simulink model "arch_logical"  (R2026a)
settings: Solver=daessc  MaxStep=MCU_Ts_FOC  RelTol=0.01
undefined symbols (not defined in the file): MCU_Ts_FOC, Param_SigProcessing_SpeedMeas_Delays, Req_Caps_Motor_Currents, Req_Caps_Motor_Torques, Req_Caps_Motor_Velocity, Req_Caps_Transmission_Torques, Req_Caps_Transmission_Velocity
libraries: simulink x5, mcbpositiondecoderlib x1
(part 1 of 2)
settings Model: DataDictionary=neck_mk3.sldd  VariantConfigurationObject=Variants  Creator=upattacini  LastModifiedBy=upattacini
settings SolverCC: MaxConsecutiveMinStep=10  SolverJacobianMethodControl=FullAnalytical  DaesscMode=Robust  ZeroCrossAlgorithm=Adaptive  DecoupledContinuousIntegration=on  MinimalZcImpactIntegration=on
settings DebuggingCC: ParameterPrecisionLossMsg=none
settings ModelReferenceCC: ModelReferenceNumInstancesAllowed=Single
settings SimscapeCC: SimscapeNominalValues="[{\"value\":\"1\",\"unit\":\"A\"},{\"value\":\"1\",\"unit\":\"bar\"},{\"value\":\"1\",\"unit\":\"cm^2\"},{\"value\":\"1\",\"unit\":\"cm^3/s\"},{\"value\":\"1\",\"unit\":\"kJ/kg\"},{\"value\":\"1\",\"unit\":\"kW\"},{\"value\":\"1\",\"unit\":\"l\"},{\"value\":\"1\",\"unit\":\"N\"},{\"value\":\"1\",\"unit\":\"N*m\"},{\"value\":\"1\",\"unit\":\"V\"}]"  SimscapeLogType=none  SimscapeLogDataHistory=5000.0
settings DiagnosticsConfigSet: SimMechanicsUnconnectedFramePorts=none
settings ExplorerConfigSet: InternalSimMechanicsExplorerSettings="<ExplorerConfiguration><canonicalview>default</canonicalview><AnimationSetting><BasePlaybackSpeed>1.0</BasePlaybackSpeed><PlaybackSpeedFactor>1.0</PlaybackSpeedFactor></AnimationSetting><TilePanel><TileInfo><Tiles Columns=\"2\" Count=\"2\" Rows=\"1\"><Column Weight=\"0.5\"/><Column Weight=\"0.5\"/><Row Weight=\"1\"/><Tile Height=\"1\" Width=\"1\" X=\"0\" Y=\"0\"/><Tile Height=\"1\" Width=\"1\" X=\"1\" Y=\"0\"/></Tiles></TileInfo><SceneInfo><SceneViewer><BGColor><R>0.60000002384185791</R><G>0.60000002384185791</G><B>0.60000002384185791</B></BGColor><Camera><DoPerspective>off</DoPerspective><Position><X>0.999998349696397781</X><Y>-0.00227288203205095948</Y><Z>0.0741295278011980668</Z></Position><Center><X>-1.65030360221862793e-06</X><Y>-0.00227288203205095948</Y><Z>0.0741295278011980668</Z></Center><Up><X>-0</X><Y>0</Y><Z>1</Z></Up><ViewLimDist>1</ViewLimDist><YLim>0.235513917526899486</YLim><XLim>0.153933287378456157</XLim></Camera></SceneViewer><SceneViewer><BGColor><R>0.60000002384185791</R><G>0.60000002384185791</G><B>0.60000002384185791</B></BGColor><Camera><DoPerspective>off</DoPerspective><Position><X>0.00315576284789383663</X><Y>0.977382858788522824</Y><Z>0.0748037208186269897</Z></Position><Center><X>0.00315576284789383663</X><Y>-0.0226171412114771764</Y><Z>0.0748037208186269897</Z></Center><Up><X>0</X><Y>0</Y><Z>1</Z></Up><ViewLimDist>1</ViewLimDist><YLim>0.228917835519784535</YLim><XLim>0.149622049223890968</XLim></Camera></SceneViewer></SceneInfo></TilePanel><MechEditorPanel><Cameras/><GfxPanelCameraMap/><VideoCreator><PlaybackSpeedRatio>1.0</PlaybackSpeedRatio><FrameRate>30</FrameRate><VideoFormat>Motion JPEG AVI</VideoFormat><FrameSize>auto</FrameSize></VideoCreator></MechEditorPanel></ExplorerConfiguration>"

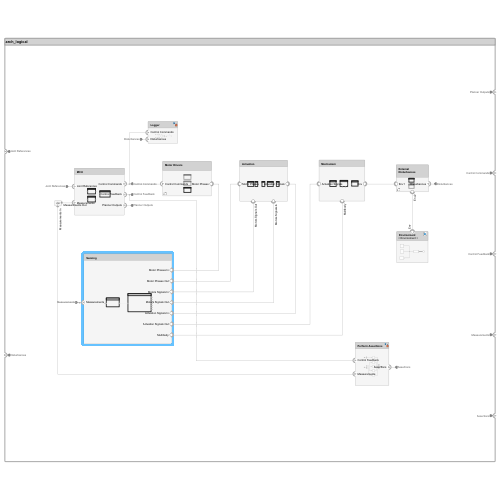
[thumbnail: Simulink's stored preview of the top-level diagram]
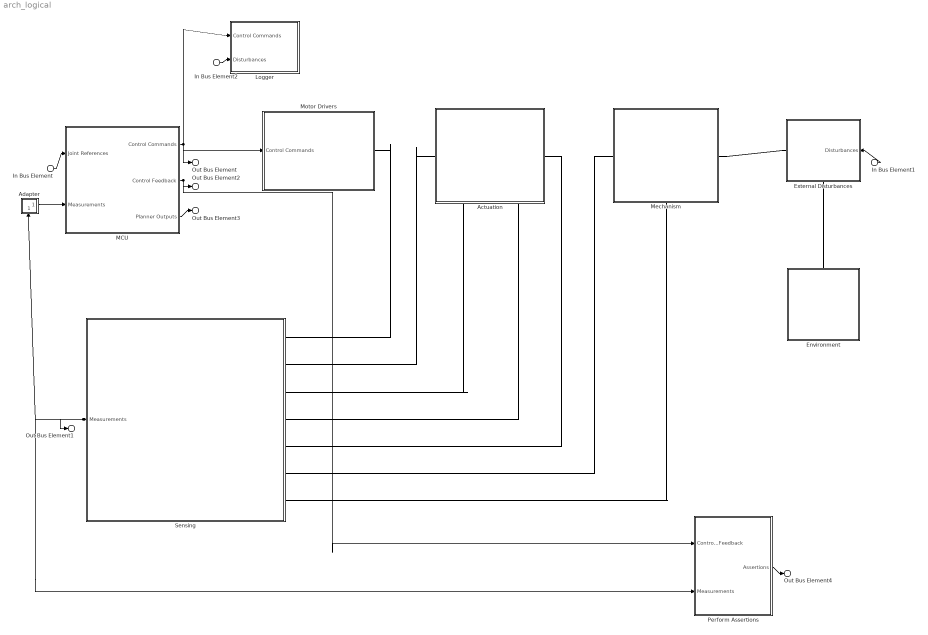
== system arch_logical ==
  In Bus Element : Inport  PortName=Joint References
  In Bus Element2 : Inport  Port=2  PortName=Disturbances
  In Bus Element1 : Inport  Port=2  PortName=Disturbances
  Actuation : Subsystem
      settings: PortSchema="{\"entries\":[{\"content\":{\"headerSize\":26,\"margin\":15,\"minimumSpacing\":25,\"sides\":[{\"content\":{\"connectorIds\":[\"LConn1\"]},\"type\":\"ConnectorPlacement.EquallySpacedRectSide\",\"uuid\":\"eccd4d58-2367-4793-bf9f-2eede0847c93\"},{\"content\":{\"connectorIds\":[\"RConn3\"],\"side\":\"RIGHT\"},\"type\":\"ConnectorPlacement.EquallySpacedRectSide\",\"uuid\":\"32519a16-e586-4f6e-b8f0-36f1e508df36\"},{\"content\":{\"side\":\"TOP\"},\"type\":\"ConnectorPlacement.EquallySpacedRectSide\",\"uuid\":\"f22ee251-d4b1-48ea-b188-f62260b2e429\"},{\"content\":{\"connectorIds\":[\"RConn1\",\"RConn2\"],\"side\":\"BOTTOM\"},\"type\":\"ConnectorPlacement.EquallySpacedRectSide\",\"uuid\":\"526c229c-fb47-4718-826e-1e8d24d62f10\"}]},\"type\":\"ConnectorPlacement.EquallySpacedConnector\",\"uuid\":\"8d6616d9-e499-47c7-92ab-9373a8f1fb5b\"}],\"packageUris\":[\"http://schema.mathworks.com/mf0/Connector/R2020b\"],\"version\":\"1.0\"}"
  Adapter : Subsystem
      settings: PortSchema="{\"entries\":[{\"content\":{\"margin\":10,\"minimumSpacing\":15,\"sides\":[{\"content\":{},\"type\":\"ConnectorPlacement.EquallySpacedRectSide\",\"uuid\":\"ddd4e9b8-61d2-4d2f-82f8-4b0ccee7ff86\"},{\"content\":{\"connectorIds\":[\"Out1\"],\"side\":\"RIGHT\"},\"type\":\"ConnectorPlacement.EquallySpacedRectSide\",\"uuid\":\"7aa9bec1-fa2e-43ed-a75e-8dec1bc414b1\"},{\"content\":{\"side\":\"TOP\"},\"type\":\"ConnectorPlacement.EquallySpacedRectSide\",\"uuid\":\"a4e0208d-8216-4c26-9a59-98a3849d45ff\"},{\"content\":{\"connectorIds\":[\"In1\"],\"side\":\"BOTTOM\"},\"type\":\"ConnectorPlacement.EquallySpacedRectSide\",\"uuid\":\"a15e082b-a01d-4828-9d21-fe1df5f3113b\"}]},\"type\":\"ConnectorPlacement.EquallySpacedConnector\",\"uuid\":\"30f7c310-01d9-4c2d-9621-d27ea52d4869\"}],\"packageUris\":[\"http://schema.mathworks.com/mf0/Connector/R2020b\"],\"version\":\"1.0\"}"
  Environment : Subsystem  ReferencedSubsystem=Environment
      settings: PermitHierarchicalResolution=None  PortSchema="{\"entries\":[{\"content\":{\"headerSize\":26,\"margin\":15,\"minimumSpacing\":25,\"sides\":[{\"content\":{},\"type\":\"ConnectorPlacement.EquallySpacedRectSide\",\"uuid\":\"f6b00979-b608-482c-ac37-5e3cc0f2d8ec\"},{\"content\":{\"side\":\"RIGHT\"},\"type\":\"ConnectorPlacement.EquallySpacedRectSide\",\"uuid\":\"5f44abf1-a2f0-4cef-bfe9-197596b0a3d4\"},{\"content\":{\"connectorIds\":[\"LConn1\"],\"side\":\"TOP\"},\"type\":\"ConnectorPlacement.EquallySpacedRectSide\",\"uuid\":\"d734854b-ebf6-45bf-86a5-9ab2f3efcb11\"}]},\"type\":\"ConnectorPlacement.EquallySpacedConnector\",\"uuid\":\"791e5e52-d9e4-45a9-9202-6f5746be1dba\"}],\"packageUris\":[\"http://schema.mathworks.com/mf0/Connector/R2020b\"],\"version\":\"1.0\"}"
  External Disturbances : Subsystem  Variant=on
      settings: PortSchema="{\"entries\":[{\"content\":{\"headerSize\":38,\"margin\":15,\"minimumSpacing\":25,\"sides\":[{\"content\":{\"connectorIds\":[\"LConn1\"]},\"type\":\"ConnectorPlacement.EquallySpacedRectSide\",\"uuid\":\"33603b70-e764-4576-b1dd-26cf30607783\"},{\"content\":{\"connectorIds\":[\"In1\"],\"side\":\"RIGHT\"},\"type\":\"ConnectorPlacement.EquallySpacedRectSide\",\"uuid\":\"a3a68558-a1a7-4632-9755-57c3560ae514\"},{\"content\":{\"side\":\"TOP\"},\"type\":\"ConnectorPlacement.EquallySpacedRectSide\",\"uuid\":\"b23d66c8-b58e-4330-a87a-a66fbfde4bac\"},{\"content\":{\"connectorIds\":[\"RConn1\"],\"side\":\"BOTTOM\"},\"type\":\"ConnectorPlacement.EquallySpacedRectSide\",\"uuid\":\"ddce90a1-93e2-4050-b1a6-c0a57aaedfd0\"}]},\"type\":\"ConnectorPlacement.EquallySpacedConnector\",\"uuid\":\"a21cd2dd-5f0f-4e3a-a097-c75bbf9b17ea\"}],\"packageUris\":[\"http://schema.mathworks.com/mf0/Connector/R2020b\"],\"version\":\"1.0\"}"
  Logger : Subsystem
      settings: PortSchema="{\"entries\":[{\"content\":{\"headerSize\":26,\"margin\":15,\"minimumSpacing\":25,\"sides\":[{\"content\":{\"connectorIds\":[\"In1\",\"In2\"]},\"type\":\"ConnectorPlacement.EquallySpacedRectSide\",\"uuid\":\"65ac2ed1-7c11-4706-b70c-547f3fcd72fb\"},{\"content\":{\"side\":\"RIGHT\"},\"type\":\"ConnectorPlacement.EquallySpacedRectSide\",\"uuid\":\"43a8be03-007c-48f6-8206-f0e589a590d5\"},{\"content\":{\"side\":\"TOP\"},\"type\":\"ConnectorPlacement.EquallySpacedRectSide\",\"uuid\":\"b148268f-cdaa-4750-84b0-59dc44f9d503\"}]},\"type\":\"ConnectorPlacement.EquallySpacedConnector\",\"uuid\":\"585a072c-b035-4c62-8ea3-f86f09820a73\"}],\"packageUris\":[\"http://schema.mathworks.com/mf0/Connector/R2020b\"],\"version\":\"1.0\"}"
  MCU : Subsystem
      settings: PortSchema="{\"entries\":[{\"content\":{\"headerSize\":26,\"margin\":15,\"minimumSpacing\":25,\"sides\":[{\"content\":{\"connectorIds\":[\"In1\",\"In2\"]},\"type\":\"ConnectorPlacement.EquallySpacedRectSide\",\"uuid\":\"b54566be-7d6a-42e3-8256-e5ad2e1ce034\"},{\"content\":{\"connectorIds\":[\"Out1\",\"Out2\",\"Out3\"],\"side\":\"RIGHT\"},\"type\":\"ConnectorPlacement.EquallySpacedRectSide\",\"uuid\":\"9e345ba6-81d0-4c80-9f55-b1ae75a52336\"},{\"content\":{\"side\":\"TOP\"},\"type\":\"ConnectorPlacement.EquallySpacedRectSide\",\"uuid\":\"65493873-4b6a-4bd2-b369-4b5afbe663c1\"}]},\"type\":\"ConnectorPlacement.EquallySpacedConnector\",\"uuid\":\"ad5ace50-4b25-45a3-978b-2fbc79f5660f\"}],\"packageUris\":[\"http://schema.mathworks.com/mf0/Connector/R2020b\"],\"version\":\"1.0\"}"
  Mechanism : Subsystem
      settings: PortSchema="{\"entries\":[{\"content\":{\"headerSize\":26,\"margin\":15,\"minimumSpacing\":25,\"sides\":[{\"content\":{\"connectorIds\":[\"LConn1\"]},\"type\":\"ConnectorPlacement.EquallySpacedRectSide\",\"uuid\":\"b54566be-7d6a-42e3-8256-e5ad2e1ce034\"},{\"content\":{\"connectorIds\":[\"RConn2\"],\"side\":\"RIGHT\"},\"type\":\"ConnectorPlacement.EquallySpacedRectSide\",\"uuid\":\"9e345ba6-81d0-4c80-9f55-b1ae75a52336\"},{\"content\":{\"side\":\"TOP\"},\"type\":\"ConnectorPlacement.EquallySpacedRectSide\",\"uuid\":\"65493873-4b6a-4bd2-b369-4b5afbe663c1\"},{\"content\":{\"connectorIds\":[\"RConn1\"],\"side\":\"BOTTOM\"},\"type\":\"ConnectorPlacement.EquallySpacedRectSide\",\"uuid\":\"11601a88-a8f5-4a5d-8ff5-68e33c191022\"}]},\"type\":\"ConnectorPlacement.EquallySpacedConnector\",\"uuid\":\"ad5ace50-4b25-45a3-978b-2fbc79f5660f\"}],\"packageUris\":[\"http://schema.mathworks.com/mf0/Connector/R2020b\"],\"version\":\"1.0\"}"
  Motor Drivers : Subsystem  Variant=on  VariantControl=Motor Drivers
      settings: PortSchema="{\"entries\":[{\"content\":{\"headerSize\":38,\"margin\":15,\"minimumSpacing\":25,\"sides\":[{\"content\":{\"connectorIds\":[\"In1\"]},\"type\":\"ConnectorPlacement.EquallySpacedRectSide\",\"uuid\":\"b54566be-7d6a-42e3-8256-e5ad2e1ce034\"},{\"content\":{\"connectorIds\":[\"RConn1\"],\"side\":\"RIGHT\"},\"type\":\"ConnectorPlacement.EquallySpacedRectSide\",\"uuid\":\"9e345ba6-81d0-4c80-9f55-b1ae75a52336\"},{\"content\":{\"side\":\"TOP\"},\"type\":\"ConnectorPlacement.EquallySpacedRectSide\",\"uuid\":\"65493873-4b6a-4bd2-b369-4b5afbe663c1\"},{\"content\":{\"side\":\"BOTTOM\"},\"type\":\"ConnectorPlacement.EquallySpacedRectSide\",\"uuid\":\"3cc66b1c-56d1-4d78-a9e5-9d06027f9ae8\"}]},\"type\":\"ConnectorPlacement.EquallySpacedConnector\",\"uuid\":\"ad5ace50-4b25-45a3-978b-2fbc79f5660f\"}],\"packageUris\":[\"http://schema.mathworks.com/mf0/Connector/R2020b\"],\"version\":\"1.0\"}"
  Perform Assertions : Subsystem
      settings: PortSchema="{\"entries\":[{\"content\":{\"headerSize\":26,\"margin\":15,\"minimumSpacing\":25,\"sides\":[{\"content\":{\"connectorIds\":[\"In1\",\"In2\"]},\"type\":\"ConnectorPlacement.EquallySpacedRectSide\",\"uuid\":\"82c0ead8-d93b-49b4-8ef2-f1de25cac233\"},{\"content\":{\"connectorIds\":[\"Out1\"],\"side\":\"RIGHT\"},\"type\":\"ConnectorPlacement.EquallySpacedRectSide\",\"uuid\":\"6d5659d8-ecac-4768-8c45-d01ff14cc080\"},{\"content\":{\"side\":\"TOP\"},\"type\":\"ConnectorPlacement.EquallySpacedRectSide\",\"uuid\":\"9d1e362c-8c75-499e-8163-f41cb6c6f816\"}]},\"type\":\"ConnectorPlacement.EquallySpacedConnector\",\"uuid\":\"50d0fcc9-d013-4bf8-8bdb-8a7263d96f85\"}],\"packageUris\":[\"http://schema.mathworks.com/mf0/Connector/R2020b\"],\"version\":\"1.0\"}"
  Sensing : Subsystem
      settings: PortSchema="{\"entries\":[{\"content\":{\"headerSize\":26,\"margin\":15,\"minimumSpacing\":25,\"sides\":[{\"content\":{\"connectorIds\":[\"Out1\"]},\"type\":\"ConnectorPlacement.EquallySpacedRectSide\",\"uuid\":\"49c15c88-294a-49d3-a3e9-7e9d2d7e0fbb\"},{\"content\":{\"connectorIds\":[\"RConn1\",\"RConn2\",\"RConn3\",\"RConn4\",\"RConn5\",\"RConn6\",\"RConn7\"],\"side\":\"RIGHT\"},\"type\":\"ConnectorPlacement.EquallySpacedRectSide\",\"uuid\":\"231f3a62-e970-4c5e-be8a-7dda6d603d83\"},{\"content\":{\"side\":\"TOP\"},\"type\":\"ConnectorPlacement.EquallySpacedRectSide\",\"uuid\":\"403ac151-60ed-4891-8e31-1a38c9d325e1\"}]},\"type\":\"ConnectorPlacement.EquallySpacedConnector\",\"uuid\":\"3d0f34fd-30d8-4e40-9b1c-23769127a566\"}],\"packageUris\":[\"http://schema.mathworks.com/mf0/Connector/R2020b\"],\"version\":\"1.0\"}"
  Out Bus Element3 : Outport  PortName=Planner Outputs
  Out Bus Element : Outport  Port=2  PortName=Control Commands
  Out Bus Element2 : Outport  Port=3  PortName=Control Feedback
  Out Bus Element1 : Outport  Port=4  PortName=Measurements
  Out Bus Element4 : Outport  Port=5  PortName=Assertions
  wires:
  MCU/1(Control Commands) -> Out Bus Element/1, Motor Drivers/1(Control Commands), Logger/1(Control Commands)
  In Bus Element/1 -> MCU/1(Joint References)
  MCU/2(Control Feedback) -> Out Bus Element2/1, Perform Assertions/1(Control Feedback)
  MCU/3(Planner Outputs) -> Out Bus Element3/1
  Perform Assertions/1(Assertions) -> Out Bus Element4/1
  Sensing/1(Measurements) -> Perform Assertions/2(Measurements), Out Bus Element1/1, Adapter/1(Measurements In)
  Adapter/1(Measurements Out) -> MCU/2(Measurements)
  In Bus Element2/1 -> Logger/2(Disturbances)
  In Bus Element1/1 -> External Disturbances/1(Disturbances)
  connections:
  Sensing/RConn1 -- Motor Drivers/RConn1
  Sensing/RConn2 -- Actuation/LConn1
  Sensing/RConn3 -- Actuation/RConn1
  Sensing/RConn4 -- Actuation/RConn2
  Sensing/RConn5 -- Actuation/RConn3
  Sensing/RConn6 -- Mechanism/LConn1
  Sensing/RConn7 -- Mechanism/RConn1
  Mechanism/RConn2 -- External Disturbances/LConn1
  Environment/LConn1 -- External Disturbances/RConn1

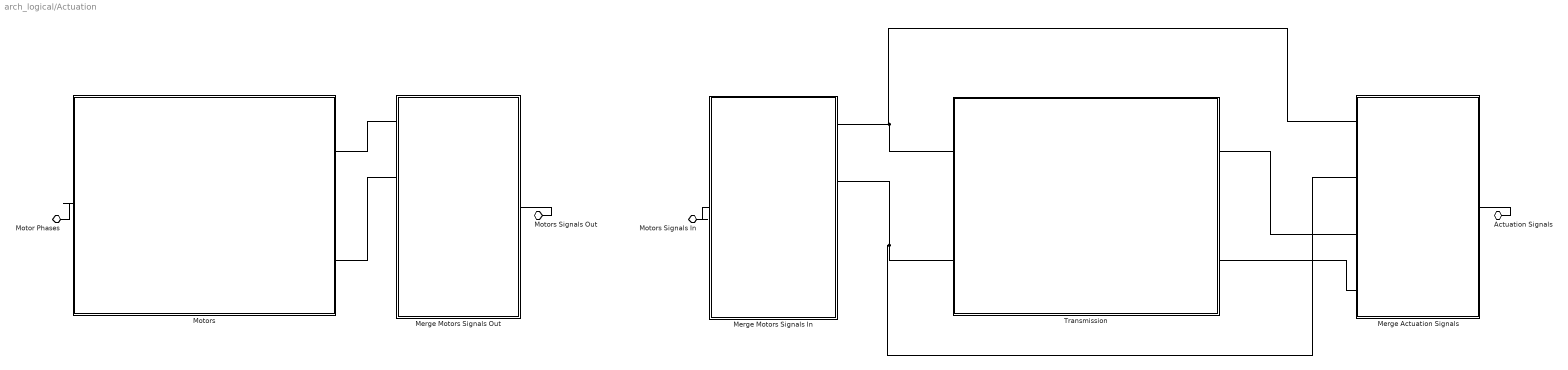
== system arch_logical/Actuation ==
  Merge Actuation Signals : Subsystem  ReferencedSubsystem=MergeActuationSignals
      settings: PermitHierarchicalResolution=None  PortSchema="{\"entries\":[{\"content\":{\"headerSize\":26,\"margin\":15,\"minimumSpacing\":25,\"sides\":[{\"content\":{\"connectorIds\":[\"LConn1\",\"LConn2\",\"LConn3\",\"LConn4\"]},\"type\":\"ConnectorPlacement.EquallySpacedRectSide\",\"uuid\":\"fc68b865-07d4-4616-83f3-8f401cbe5686\"},{\"content\":{\"connectorIds\":[\"RConn1\"],\"side\":\"RIGHT\"},\"type\":\"ConnectorPlacement.EquallySpacedRectSide\",\"uuid\":\"1658ecd9-4df8-4b52-8b24-30d2825782fa\"},{\"content\":{\"side\":\"TOP\"},\"type\":\"ConnectorPlacement.EquallySpacedRectSide\",\"uuid\":\"aa785ee9-f455-412c-96db-be9f2e01bdf6\"}]},\"type\":\"ConnectorPlacement.EquallySpacedConnector\",\"uuid\":\"1df0c366-4a53-43f1-9659-7d2b3db17667\"}],\"packageUris\":[\"http://schema.mathworks.com/mf0/Connector/R2020b\"],\"version\":\"1.0\"}"
  Merge Motors Signals In : Subsystem  ReferencedSubsystem=MergeActuationSignals
      settings: PermitHierarchicalResolution=None  PortSchema="{\"entries\":[{\"content\":{\"headerSize\":26,\"margin\":15,\"minimumSpacing\":25,\"sides\":[{\"content\":{\"connectorIds\":[\"RConn1\"]},\"type\":\"ConnectorPlacement.EquallySpacedRectSide\",\"uuid\":\"fc68b865-07d4-4616-83f3-8f401cbe5686\"},{\"content\":{\"connectorIds\":[\"LConn1\",\"LConn2\",\"LConn3\",\"LConn4\"],\"side\":\"RIGHT\"},\"type\":\"ConnectorPlacement.EquallySpacedRectSide\",\"uuid\":\"1658ecd9-4df8-4b52-8b24-30d2825782fa\"},{\"content\":{\"side\":\"TOP\"},\"type\":\"ConnectorPlacement.EquallySpacedRectSide\",\"uuid\":\"aa785ee9-f455-412c-96db-be9f2e01bdf6\"}]},\"type\":\"ConnectorPlacement.EquallySpacedConnector\",\"uuid\":\"1df0c366-4a53-43f1-9659-7d2b3db17667\"}],\"packageUris\":[\"http://schema.mathworks.com/mf0/Connector/R2020b\"],\"version\":\"1.0\"}"
  Merge Motors Signals Out : Subsystem  ReferencedSubsystem=MergeActuationSignals
      settings: PermitHierarchicalResolution=None  PortSchema="{\"entries\":[{\"content\":{\"headerSize\":26,\"margin\":15,\"minimumSpacing\":25,\"sides\":[{\"content\":{\"connectorIds\":[\"LConn1\",\"LConn2\",\"LConn3\",\"LConn4\"]},\"type\":\"ConnectorPlacement.EquallySpacedRectSide\",\"uuid\":\"fc68b865-07d4-4616-83f3-8f401cbe5686\"},{\"content\":{\"connectorIds\":[\"RConn1\"],\"side\":\"RIGHT\"},\"type\":\"ConnectorPlacement.EquallySpacedRectSide\",\"uuid\":\"1658ecd9-4df8-4b52-8b24-30d2825782fa\"},{\"content\":{\"side\":\"TOP\"},\"type\":\"ConnectorPlacement.EquallySpacedRectSide\",\"uuid\":\"aa785ee9-f455-412c-96db-be9f2e01bdf6\"}]},\"type\":\"ConnectorPlacement.EquallySpacedConnector\",\"uuid\":\"1df0c366-4a53-43f1-9659-7d2b3db17667\"}],\"packageUris\":[\"http://schema.mathworks.com/mf0/Connector/R2020b\"],\"version\":\"1.0\"}"
  Motors : Subsystem  Variant=on  VariantControl=Motors
      settings: PortSchema="{\"entries\":[{\"content\":{\"headerSize\":38,\"margin\":15,\"minimumSpacing\":25,\"sides\":[{\"content\":{\"connectorIds\":[\"LConn1\"]},\"type\":\"ConnectorPlacement.EquallySpacedRectSide\",\"uuid\":\"eccd4d58-2367-4793-bf9f-2eede0847c93\"},{\"content\":{\"connectorIds\":[\"RConn1\",\"RConn2\"],\"side\":\"RIGHT\"},\"type\":\"ConnectorPlacement.EquallySpacedRectSide\",\"uuid\":\"32519a16-e586-4f6e-b8f0-36f1e508df36\"},{\"content\":{\"side\":\"TOP\"},\"type\":\"ConnectorPlacement.EquallySpacedRectSide\",\"uuid\":\"f22ee251-d4b1-48ea-b188-f62260b2e429\"}]},\"type\":\"ConnectorPlacement.EquallySpacedConnector\",\"uuid\":\"8d6616d9-e499-47c7-92ab-9373a8f1fb5b\"}],\"packageUris\":[\"http://schema.mathworks.com/mf0/Connector/R2020b\"],\"version\":\"1.0\"}"
  Transmission : Subsystem  Variant=on  VariantControl=Transmission
      settings: PortSchema="{\"entries\":[{\"content\":{\"headerSize\":38,\"margin\":15,\"minimumSpacing\":25,\"sides\":[{\"content\":{\"connectorIds\":[\"LConn1\",\"LConn2\"]},\"type\":\"ConnectorPlacement.EquallySpacedRectSide\",\"uuid\":\"eccd4d58-2367-4793-bf9f-2eede0847c93\"},{\"content\":{\"connectorIds\":[\"RConn1\",\"RConn2\"],\"side\":\"RIGHT\"},\"type\":\"ConnectorPlacement.EquallySpacedRectSide\",\"uuid\":\"32519a16-e586-4f6e-b8f0-36f1e508df36\"},{\"content\":{\"side\":\"TOP\"},\"type\":\"ConnectorPlacement.EquallySpacedRectSide\",\"uuid\":\"f22ee251-d4b1-48ea-b188-f62260b2e429\"}]},\"type\":\"ConnectorPlacement.EquallySpacedConnector\",\"uuid\":\"8d6616d9-e499-47c7-92ab-9373a8f1fb5b\"}],\"packageUris\":[\"http://schema.mathworks.com/mf0/Connector/R2020b\"],\"version\":\"1.0\"}"
  Motor Phases : PMIOPort  Side=Left  ConnectionType=Bus: Physical_MotorPhases
  Motors Signals Out : PMIOPort  Port=2  Side=Right  ConnectionType=Bus: Physical_Actuation
  Motors Signals In : PMIOPort  Port=3  Side=Right  ConnectionType=Bus: Physical_Actuation
  Actuation Signals : PMIOPort  Port=4  Side=Right  ConnectionType=Bus: Physical_Actuation
  connections:
  Motors/LConn1 -- Motor Phases/RConn1
  Merge Actuation Signals/RConn1 -- Actuation Signals/RConn1
  Merge Actuation Signals/LConn3 -- Transmission/RConn1
  Merge Actuation Signals/LConn4 -- Transmission/RConn2
  Motors/RConn1 -- Merge Motors Signals Out/LConn1
  Motors/RConn2 -- Merge Motors Signals Out/LConn2
  Merge Motors Signals In/LConn1 -- Merge Actuation Signals/LConn1 -- Transmission/LConn1
  Merge Motors Signals In/LConn2 -- Merge Actuation Signals/LConn2 -- Transmission/LConn2
  Merge Motors Signals Out/RConn1 -- Motors Signals Out/RConn1
  Motors Signals In/RConn1 -- Merge Motors Signals In/RConn1

== system arch_logical/Adapter ==
  In Bus Element : Inport  PortName=Measurements In
  Out Bus Element : Outport  PortName=Measurements Out
  wires:
  In Bus Element/1 -> Out Bus Element/1

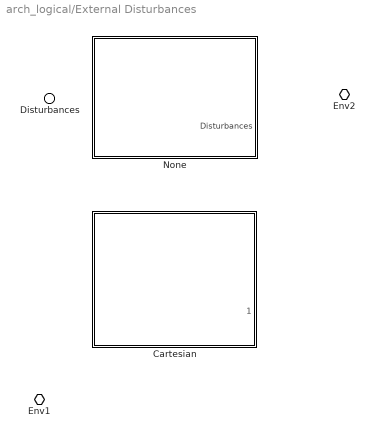
== system arch_logical/External Disturbances ==
  Disturbances : Inport  OutDataTypeStr=Bus: Data_Disturbances
  Cartesian : Subsystem  VariantControl=Selector_Disturbances == Types_Disturbances.Cartesian  ReferencedSubsystem=Disturbances_Cartesian
      settings: PermitHierarchicalResolution=None  PortSchema="{\"entries\":[{\"content\":{\"headerSize\":26,\"margin\":15,\"minimumSpacing\":25,\"sides\":[{\"content\":{\"connectorIds\":[\"LConn1\"]},\"type\":\"ConnectorPlacement.EquallySpacedRectSide\",\"uuid\":\"7de4a9b9-1c78-468b-b31f-7d9f33f70814\"},{\"content\":{\"connectorIds\":[\"RConn1\",\"In1\"],\"side\":\"RIGHT\"},\"type\":\"ConnectorPlacement.EquallySpacedRectSide\",\"uuid\":\"cb72d83b-da52-42c4-b541-8abbb9837007\"},{\"content\":{\"side\":\"TOP\"},\"type\":\"ConnectorPlacement.EquallySpacedRectSide\",\"uuid\":\"2fe19e56-7f0b-493f-96d4-9ec1fff1add0\"},{\"content\":{\"side\":\"BOTTOM\"},\"type\":\"ConnectorPlacement.EquallySpacedRectSide\",\"uuid\":\"ba0fcf55-7e24-4730-939f-0caa7aae1ac9\"}]},\"type\":\"ConnectorPlacement.EquallySpacedConnector\",\"uuid\":\"d29630cb-5feb-4771-95d4-59cb3f7fb024\"}],\"packageUris\":[\"http://schema.mathworks.com/mf0/Connector/R2020b\"],\"version\":\"1.0\"}"
  None : Subsystem  VariantControl=Selector_Disturbances == Types_Disturbances.None
      settings: PortSchema="{\"entries\":[{\"content\":{\"headerSize\":26,\"margin\":15,\"minimumSpacing\":25,\"sides\":[{\"content\":{\"connectorIds\":[\"LConn1\"]},\"type\":\"ConnectorPlacement.EquallySpacedRectSide\",\"uuid\":\"7de4a9b9-1c78-468b-b31f-7d9f33f70814\"},{\"content\":{\"connectorIds\":[\"RConn1\",\"In1\"],\"side\":\"RIGHT\"},\"type\":\"ConnectorPlacement.EquallySpacedRectSide\",\"uuid\":\"cb72d83b-da52-42c4-b541-8abbb9837007\"},{\"content\":{\"side\":\"TOP\"},\"type\":\"ConnectorPlacement.EquallySpacedRectSide\",\"uuid\":\"2fe19e56-7f0b-493f-96d4-9ec1fff1add0\"},{\"content\":{\"side\":\"BOTTOM\"},\"type\":\"ConnectorPlacement.EquallySpacedRectSide\",\"uuid\":\"3d6aa6e6-fd5d-4623-92b1-ca6cfa3cb9de\"}]},\"type\":\"ConnectorPlacement.EquallySpacedConnector\",\"uuid\":\"d29630cb-5feb-4771-95d4-59cb3f7fb024\"}],\"packageUris\":[\"http://schema.mathworks.com/mf0/Connector/R2020b\"],\"version\":\"1.0\"}"
  Env1 : PMIOPort  Side=Left
  Env2 : PMIOPort  Port=2  Side=Right

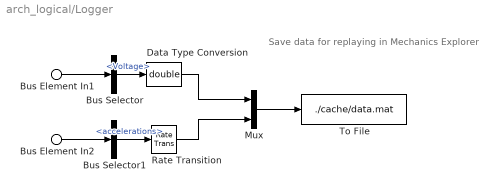
== system arch_logical/Logger ==
  note: Save data for replaying in Mechanics Explorer
  Bus Element In1 : Inport  PortName=Control Commands
  Bus Element In2 : Inport  Port=2  PortName=Disturbances
  Bus Selector : BusSelector  OutputSignals=Voltage
  Bus Selector1 : BusSelector  OutputSignals=accelerations
  Data Type Conversion : DataTypeConversion  OutDataTypeStr=double  SaturateOnIntegerOverflow=off  RndMeth=Floor
  Mux : Mux  Inputs=2
  Rate Transition : RateTransition  Deterministic=off
  To File : ToFile  Filename=./cache/data.mat  MatrixName=data  SaveFormat=Timeseries  SampleTime=MCU_Ts_FOC
  wires:
  Bus Element In1/1 -> Bus Selector/1
  Bus Selector/1 -> Data Type Conversion/1  "<Voltage>"
  Bus Selector1/1 -> Rate Transition/1  "<accelerations>"
  Mux/1 -> To File/1
  Data Type Conversion/1 -> Mux/1
  Bus Element In2/1 -> Bus Selector1/1
  Rate Transition/1 -> Mux/2

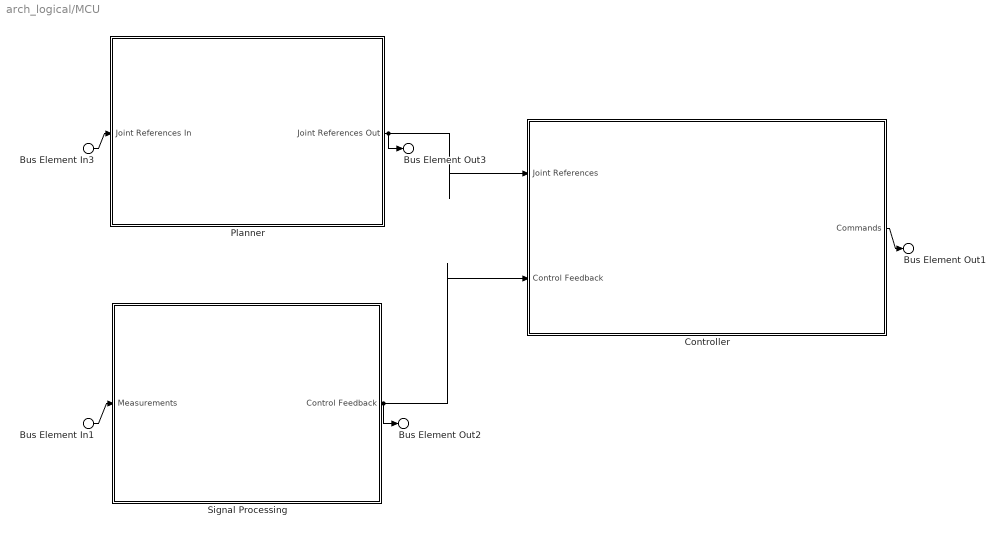
== system arch_logical/MCU ==
  Bus Element In3 : Inport  PortName=Joint References
  Bus Element In1 : Inport  Port=2  PortName=Measurements
  Controller : Subsystem  Variant=on  VariantControl=Controller
      settings: PortSchema="{\"entries\":[{\"content\":{\"headerSize\":38,\"margin\":15,\"minimumSpacing\":25,\"sides\":[{\"content\":{\"connectorIds\":[\"In1\",\"In2\"]},\"type\":\"ConnectorPlacement.EquallySpacedRectSide\",\"uuid\":\"b54566be-7d6a-42e3-8256-e5ad2e1ce034\"},{\"content\":{\"connectorIds\":[\"Out1\"],\"side\":\"RIGHT\"},\"type\":\"ConnectorPlacement.EquallySpacedRectSide\",\"uuid\":\"9e345ba6-81d0-4c80-9f55-b1ae75a52336\"},{\"content\":{\"side\":\"TOP\"},\"type\":\"ConnectorPlacement.EquallySpacedRectSide\",\"uuid\":\"65493873-4b6a-4bd2-b369-4b5afbe663c1\"}]},\"type\":\"ConnectorPlacement.EquallySpacedConnector\",\"uuid\":\"ad5ace50-4b25-45a3-978b-2fbc79f5660f\"}],\"packageUris\":[\"http://schema.mathworks.com/mf0/Connector/R2020b\"],\"version\":\"1.0\"}"
  Planner : Subsystem  Variant=on  VariantControl=Planner
      settings: PortSchema="{\"entries\":[{\"content\":{\"headerSize\":38,\"margin\":15,\"minimumSpacing\":25,\"sides\":[{\"content\":{\"connectorIds\":[\"In1\"]},\"type\":\"ConnectorPlacement.EquallySpacedRectSide\",\"uuid\":\"4dcdf3d9-66d1-4b2d-9c68-f21e4e282afd\"},{\"content\":{\"connectorIds\":[\"Out1\"],\"side\":\"RIGHT\"},\"type\":\"ConnectorPlacement.EquallySpacedRectSide\",\"uuid\":\"3179edab-f19d-4e86-a6d0-5fab8993b041\"},{\"content\":{\"side\":\"TOP\"},\"type\":\"ConnectorPlacement.EquallySpacedRectSide\",\"uuid\":\"71bb34ca-738a-4841-9245-23739004f511\"}]},\"type\":\"ConnectorPlacement.EquallySpacedConnector\",\"uuid\":\"4120f61b-053a-45ce-ab11-ff3b69017e22\"}],\"packageUris\":[\"http://schema.mathworks.com/mf0/Connector/R2020b\"],\"version\":\"1.0\"}"
  Signal Processing : Subsystem  Variant=on  VariantControl=Signal Processing
      settings: PortSchema="{\"entries\":[{\"content\":{\"headerSize\":38,\"margin\":15,\"minimumSpacing\":25,\"sides\":[{\"content\":{\"connectorIds\":[\"In1\"]},\"type\":\"ConnectorPlacement.EquallySpacedRectSide\",\"uuid\":\"eccd4d58-2367-4793-bf9f-2eede0847c93\"},{\"content\":{\"connectorIds\":[\"Out1\"],\"side\":\"RIGHT\"},\"type\":\"ConnectorPlacement.EquallySpacedRectSide\",\"uuid\":\"32519a16-e586-4f6e-b8f0-36f1e508df36\"},{\"content\":{\"side\":\"TOP\"},\"type\":\"ConnectorPlacement.EquallySpacedRectSide\",\"uuid\":\"f22ee251-d4b1-48ea-b188-f62260b2e429\"},{\"content\":{\"side\":\"BOTTOM\"},\"type\":\"ConnectorPlacement.EquallySpacedRectSide\",\"uuid\":\"044c0013-73b4-4eb7-b0dc-011a4b3384d3\"}]},\"type\":\"ConnectorPlacement.EquallySpacedConnector\",\"uuid\":\"8d6616d9-e499-47c7-92ab-9373a8f1fb5b\"}],\"packageUris\":[\"http://schema.mathworks.com/mf0/Connector/R2020b\"],\"version\":\"1.0\"}"
  Bus Element Out1 : Outport  PortName=Control Commands
  Bus Element Out2 : Outport  Port=2  PortName=Control Feedback
  Bus Element Out3 : Outport  Port=3  PortName=Planner Outputs
  wires:
  Controller/1(Commands) -> Bus Element Out1/1
  Bus Element In3/1 -> Planner/1(Joint References In)
  Planner/1(Joint References Out) -> Bus Element Out3/1, Controller/1(Joint References)
  Bus Element In1/1 -> Signal Processing/1(Measurements)
  Signal Processing/1(Control Feedback) -> Bus Element Out2/1, Controller/2(Control Feedback)

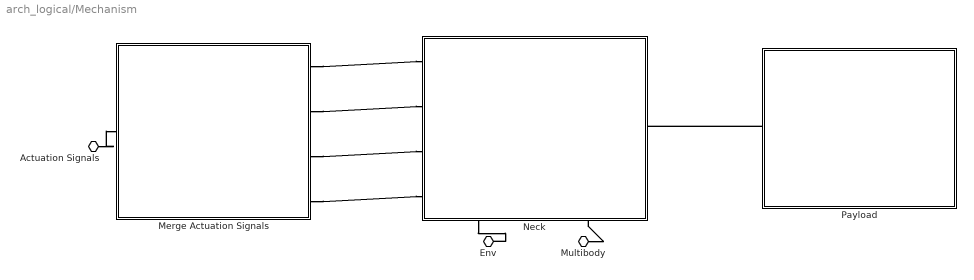
== system arch_logical/Mechanism ==
  Merge Actuation Signals : Subsystem  ReferencedSubsystem=MergeActuationSignals
      settings: PermitHierarchicalResolution=None  PortSchema="{\"entries\":[{\"content\":{\"headerSize\":26,\"margin\":15,\"minimumSpacing\":25,\"sides\":[{\"content\":{\"connectorIds\":[\"RConn1\"]},\"type\":\"ConnectorPlacement.EquallySpacedRectSide\",\"uuid\":\"fc68b865-07d4-4616-83f3-8f401cbe5686\"},{\"content\":{\"connectorIds\":[\"LConn1\",\"LConn2\",\"LConn3\",\"LConn4\"],\"side\":\"RIGHT\"},\"type\":\"ConnectorPlacement.EquallySpacedRectSide\",\"uuid\":\"1658ecd9-4df8-4b52-8b24-30d2825782fa\"},{\"content\":{\"side\":\"TOP\"},\"type\":\"ConnectorPlacement.EquallySpacedRectSide\",\"uuid\":\"aa785ee9-f455-412c-96db-be9f2e01bdf6\"}]},\"type\":\"ConnectorPlacement.EquallySpacedConnector\",\"uuid\":\"1df0c366-4a53-43f1-9659-7d2b3db17667\"}],\"packageUris\":[\"http://schema.mathworks.com/mf0/Connector/R2020b\"],\"version\":\"1.0\"}"
  Neck : Subsystem  Variant=on  VariantControl=Neck
      settings: PortSchema="{\"entries\":[{\"content\":{\"headerSize\":38,\"margin\":15,\"minimumSpacing\":25,\"sides\":[{\"content\":{\"connectorIds\":[\"LConn1\",\"LConn2\",\"LConn3\",\"LConn4\"]},\"type\":\"ConnectorPlacement.EquallySpacedRectSide\",\"uuid\":\"57d6c408-3008-4772-82fa-c78950aeb972\"},{\"content\":{\"connectorIds\":[\"RConn1\"],\"side\":\"RIGHT\"},\"type\":\"ConnectorPlacement.EquallySpacedRectSide\",\"uuid\":\"be30f5ae-b864-4f0d-80fa-3961a8cb329f\"},{\"content\":{\"side\":\"TOP\"},\"type\":\"ConnectorPlacement.EquallySpacedRectSide\",\"uuid\":\"34d93d68-430e-44f9-8eee-ecae2c4e1418\"},{\"content\":{\"connectorIds\":[\"RConn3\",\"RConn2\"],\"side\":\"BOTTOM\"},\"type\":\"ConnectorPlacement.EquallySpacedRectSide\",\"uuid\":\"c172c7ca-a849-4a61-b14b-b119063e659c\"}]},\"type\":\"ConnectorPlacement.EquallySpacedConnector\",\"uuid\":\"47a4edbe-a09b-4305-8f4f-fa3fc9056d60\"}],\"packageUris\":[\"http://schema.mathworks.com/mf0/Connector/R2020b\"],\"version\":\"1.0\"}"
  Payload : Subsystem  Variant=on  VariantControl=Payload
      settings: PortSchema="{\"entries\":[{\"content\":{\"headerSize\":38,\"margin\":15,\"minimumSpacing\":25,\"sides\":[{\"content\":{\"connectorIds\":[\"LConn1\"]},\"type\":\"ConnectorPlacement.EquallySpacedRectSide\",\"uuid\":\"57d6c408-3008-4772-82fa-c78950aeb972\"},{\"content\":{\"side\":\"RIGHT\"},\"type\":\"ConnectorPlacement.EquallySpacedRectSide\",\"uuid\":\"be30f5ae-b864-4f0d-80fa-3961a8cb329f\"},{\"content\":{\"side\":\"TOP\"},\"type\":\"ConnectorPlacement.EquallySpacedRectSide\",\"uuid\":\"34d93d68-430e-44f9-8eee-ecae2c4e1418\"}]},\"type\":\"ConnectorPlacement.EquallySpacedConnector\",\"uuid\":\"47a4edbe-a09b-4305-8f4f-fa3fc9056d60\"}],\"packageUris\":[\"http://schema.mathworks.com/mf0/Connector/R2020b\"],\"version\":\"1.0\"}"
  Multibody : PMIOPort  Side=Right  ConnectionType=Bus: Physical_Multibody
  Env : PMIOPort  Port=2  Side=Right  ConnectionType=Bus: Physical_Environment
  Actuation Signals : PMIOPort  Port=3  Side=Left  ConnectionType=Bus: Physical_Actuation
  connections:
  Neck/RConn3 -- Env/RConn1
  Payload/LConn1 -- Neck/RConn1
  Multibody/RConn1 -- Neck/RConn2
  Actuation Signals/RConn1 -- Merge Actuation Signals/RConn1
  Merge Actuation Signals/LConn1 -- Neck/LConn1
  Merge Actuation Signals/LConn2 -- Neck/LConn2
  Merge Actuation Signals/LConn3 -- Neck/LConn3
  Merge Actuation Signals/LConn4 -- Neck/LConn4

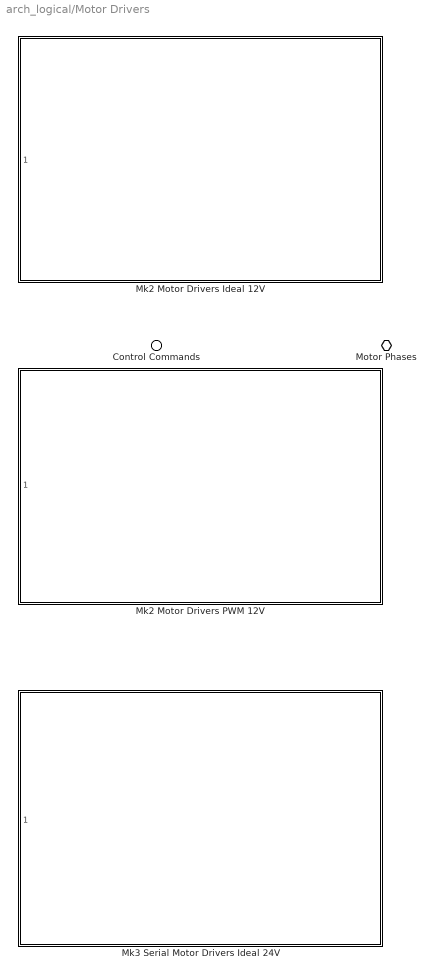
== system arch_logical/Motor Drivers ==
  Control Commands : Inport  OutDataTypeStr=Bus: Data_ControlCommands
  Mk2 Motor Drivers Ideal 12V : Subsystem  VariantControl=Selector_MotorDriver == Types_MotorDriver.DC_Ideal_12V  ReferencedSubsystem=Mk2MotorDrivers_Ideal
      settings: PermitHierarchicalResolution=None  PortSchema="{\"entries\":[{\"content\":{\"headerSize\":26,\"margin\":15,\"minimumSpacing\":25,\"sides\":[{\"content\":{\"connectorIds\":[\"In1\"]},\"type\":\"ConnectorPlacement.EquallySpacedRectSide\",\"uuid\":\"c3450419-cf63-43fd-b34e-462186fbc4d5\"},{\"content\":{\"connectorIds\":[\"RConn1\"],\"side\":\"RIGHT\"},\"type\":\"ConnectorPlacement.EquallySpacedRectSide\",\"uuid\":\"72941fe2-1c11-4054-ae77-a46e9405913a\"},{\"content\":{\"side\":\"TOP\"},\"type\":\"ConnectorPlacement.EquallySpacedRectSide\",\"uuid\":\"3371313f-8ed2-4a14-9ef4-fd010c7033a0\"}]},\"type\":\"ConnectorPlacement.EquallySpacedConnector\",\"uuid\":\"aa89ab5c-df29-4a6e-9b3a-4709c266d048\"}],\"packageUris\":[\"http://schema.mathworks.com/mf0/Connector/R2020b\"],\"version\":\"1.0\"}"
  Mk2 Motor Drivers PWM 12V : Subsystem  VariantControl=Selector_MotorDriver == Types_MotorDriver.DC_PWM_12V  ReferencedSubsystem=Mk2MotorDrivers_PWM
      settings: PermitHierarchicalResolution=None  PortSchema="{\"entries\":[{\"content\":{\"headerSize\":26,\"margin\":15,\"minimumSpacing\":25,\"sides\":[{\"content\":{\"connectorIds\":[\"In1\"]},\"type\":\"ConnectorPlacement.EquallySpacedRectSide\",\"uuid\":\"c3450419-cf63-43fd-b34e-462186fbc4d5\"},{\"content\":{\"connectorIds\":[\"RConn1\"],\"side\":\"RIGHT\"},\"type\":\"ConnectorPlacement.EquallySpacedRectSide\",\"uuid\":\"72941fe2-1c11-4054-ae77-a46e9405913a\"},{\"content\":{\"side\":\"TOP\"},\"type\":\"ConnectorPlacement.EquallySpacedRectSide\",\"uuid\":\"3371313f-8ed2-4a14-9ef4-fd010c7033a0\"}]},\"type\":\"ConnectorPlacement.EquallySpacedConnector\",\"uuid\":\"aa89ab5c-df29-4a6e-9b3a-4709c266d048\"}],\"packageUris\":[\"http://schema.mathworks.com/mf0/Connector/R2020b\"],\"version\":\"1.0\"}"
  Mk3 Serial Motor Drivers Ideal 24V : Subsystem  VariantControl=Selector_MotorDriver == Types_MotorDriver.DC_Ideal_24V  ReferencedSubsystem=Mk3SerialMotorDrivers_Ideal
      settings: PermitHierarchicalResolution=None  PortSchema="{\"entries\":[{\"content\":{\"headerSize\":26,\"margin\":15,\"minimumSpacing\":25,\"sides\":[{\"content\":{\"connectorIds\":[\"In1\"]},\"type\":\"ConnectorPlacement.EquallySpacedRectSide\",\"uuid\":\"25b65f7d-f824-4ba3-b1ed-62665898e2af\"},{\"content\":{\"connectorIds\":[\"RConn1\"],\"side\":\"RIGHT\"},\"type\":\"ConnectorPlacement.EquallySpacedRectSide\",\"uuid\":\"9487a21d-3ba6-4fe2-bdba-f10d1b29e9d5\"},{\"content\":{\"side\":\"TOP\"},\"type\":\"ConnectorPlacement.EquallySpacedRectSide\",\"uuid\":\"4746a095-1b27-40e2-b199-adb40e90c46e\"}]},\"type\":\"ConnectorPlacement.EquallySpacedConnector\",\"uuid\":\"2d26b106-d6e1-4bff-b1c2-31dab5640331\"}],\"packageUris\":[\"http://schema.mathworks.com/mf0/Connector/R2020b\"],\"version\":\"1.0\"}"
  Motor Phases : PMIOPort  Side=Right  ConnectionType=Bus: Physical_MotorPhases

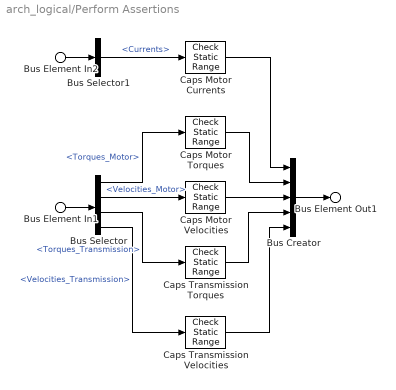
== system arch_logical/Perform Assertions ==
  Bus Element In2 : Inport  PortName=Control Feedback
  Bus Element In1 : Inport  Port=2  PortName=Measurements
  Bus Creator : BusCreator  Inputs=5  OutDataTypeStr=Bus: Data_Assertions  NonVirtualBus=on
      settings: InheritFromInputs=off
  Bus Selector : BusSelector  OutputSignals=Torques_Motor,Velocities_Motor,Torques_Transmission,Velocities_Transmission
  Bus Selector1 : BusSelector  OutputSignals=Currents
  Caps Motor Currents : simulink/Model Verification/Check  Static Range  Description=-Req_Caps_Motor_Currents <= u <= Req_Caps_Motor_Currents  max=Req_Caps_Motor_Currents  max_included=on  min=-Req_Caps_Motor_Currents  min_included=on  enabled=on  stopWhenAssertionFail=off  export=on  icon=graphic
  Caps Motor Torques : simulink/Model Verification/Check  Static Range  Description=-Req_Caps_Motor_Torques <= u <= Req_Caps_Motor_Torques  max=Req_Caps_Motor_Torques  max_included=on  min=-Req_Caps_Motor_Torques  min_included=on  enabled=on  stopWhenAssertionFail=off  export=on  icon=graphic
  Caps Motor Velocities : simulink/Model Verification/Check  Static Range  Description=-Req_Caps_Motor_Velocity <= u <= Req_Caps_Motor_Velocity  max=Req_Caps_Motor_Velocity  max_included=on  min=-Req_Caps_Motor_Velocity  min_included=on  enabled=on  stopWhenAssertionFail=off  export=on  icon=graphic
  Caps Transmission Torques : simulink/Model Verification/Check  Static Range  Description=-Req_Caps_Transmission_Torques <= u <= Req_Caps_Transmission_Torques  max=Req_Caps_Transmission_Torques  max_included=on  min=-Req_Caps_Transmission_Torques  min_included=on  enabled=on  stopWhenAssertionFail=off  export=on  icon=graphic
  Caps Transmission Velocities : simulink/Model Verification/Check  Static Range  Description=-Req_Caps_Transmission_Velocity <= u <= Req_Caps_Transmission_Velocity  max=Req_Caps_Transmission_Velocity  max_included=on  min=-Req_Caps_Transmission_Velocity  min_included=on  enabled=on  stopWhenAssertionFail=off  export=on  icon=graphic
  Bus Element Out1 : Outport  PortName=Assertions
  wires:
  Bus Element In1/1 -> Bus Selector/1
  Bus Selector/1 -> Caps Motor Torques/1  "<Torques_Motor>"
  Bus Selector/2 -> Caps Motor Velocities/1  "<Velocities_Motor>"
  Bus Selector/3 -> Caps Transmission Torques/1  "<Torques_Transmission>"
  Bus Selector/4 -> Caps Transmission Velocities/1  "<Velocities_Transmission>"
  Bus Element In2/1 -> Bus Selector1/1
  Bus Selector1/1 -> Caps Motor Currents/1  "<Currents>"
  Bus Creator/1 -> Bus Element Out1/1
  Caps Motor Currents/1 -> Bus Creator/1
  Caps Motor Torques/1 -> Bus Creator/2
  Caps Motor Velocities/1 -> Bus Creator/3
  Caps Transmission Torques/1 -> Bus Creator/4
  Caps Transmission Velocities/1 -> Bus Creator/5

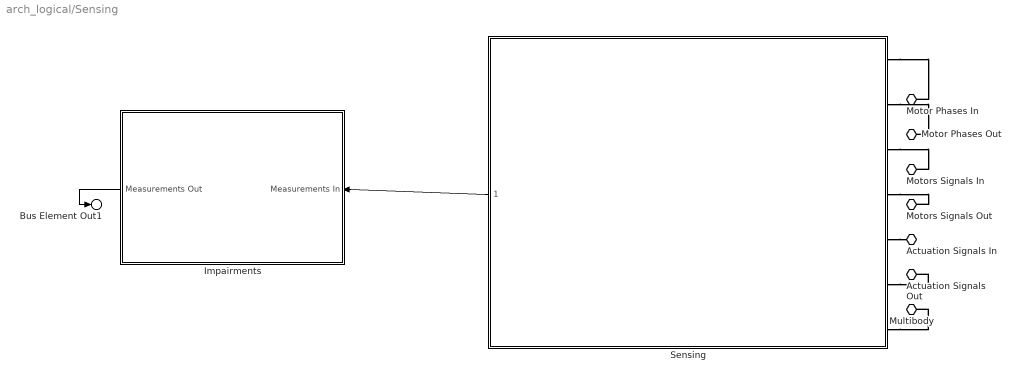
== system arch_logical/Sensing ==
  Impairments : Subsystem  Variant=on
      settings: PortSchema="{\"entries\":[{\"content\":{\"headerSize\":38,\"margin\":15,\"minimumSpacing\":25,\"sides\":[{\"content\":{\"connectorIds\":[\"Out1\"]},\"type\":\"ConnectorPlacement.EquallySpacedRectSide\",\"uuid\":\"87e5b18e-a8fb-4e72-a16b-0f3a4065fd11\"},{\"content\":{\"connectorIds\":[\"In1\"],\"side\":\"RIGHT\"},\"type\":\"ConnectorPlacement.EquallySpacedRectSide\",\"uuid\":\"56c0bf66-4087-46b6-8583-60f74a03dd55\"},{\"content\":{\"side\":\"TOP\"},\"type\":\"ConnectorPlacement.EquallySpacedRectSide\",\"uuid\":\"6d44a9d6-c3ee-43e7-b2a9-4c5a4c110eca\"}]},\"type\":\"ConnectorPlacement.EquallySpacedConnector\",\"uuid\":\"7c2b7503-7794-4170-aa8c-71ff6331f431\"}],\"packageUris\":[\"http://schema.mathworks.com/mf0/Connector/R2020b\"],\"version\":\"1.0\"}"
  Sensing : Subsystem  ReferencedSubsystem=Sensing
      settings: PermitHierarchicalResolution=None  PortSchema="{\"entries\":[{\"content\":{\"headerSize\":26,\"margin\":15,\"minimumSpacing\":25,\"sides\":[{\"content\":{\"connectorIds\":[\"Out1\"]},\"type\":\"ConnectorPlacement.EquallySpacedRectSide\",\"uuid\":\"49c15c88-294a-49d3-a3e9-7e9d2d7e0fbb\"},{\"content\":{\"connectorIds\":[\"RConn1\",\"RConn2\",\"RConn3\",\"RConn4\",\"RConn5\",\"RConn6\",\"RConn7\"],\"side\":\"RIGHT\"},\"type\":\"ConnectorPlacement.EquallySpacedRectSide\",\"uuid\":\"231f3a62-e970-4c5e-be8a-7dda6d603d83\"},{\"content\":{\"side\":\"TOP\"},\"type\":\"ConnectorPlacement.EquallySpacedRectSide\",\"uuid\":\"403ac151-60ed-4891-8e31-1a38c9d325e1\"}]},\"type\":\"ConnectorPlacement.EquallySpacedConnector\",\"uuid\":\"3d0f34fd-30d8-4e40-9b1c-23769127a566\"}],\"packageUris\":[\"http://schema.mathworks.com/mf0/Connector/R2020b\"],\"version\":\"1.0\"}"
  Motor Phases In : PMIOPort  Side=Right  ConnectionType=Bus: Physical_MotorPhases
  Motor Phases Out : PMIOPort  Port=2  Side=Right  ConnectionType=Bus: Physical_MotorPhases
  Motors Signals In : PMIOPort  Port=3  Side=Right  ConnectionType=Bus: Physical_Actuation
  Motors Signals Out : PMIOPort  Port=4  Side=Right  ConnectionType=Bus: Physical_Actuation
  Actuation Signals In : PMIOPort  Port=5  Side=Right  ConnectionType=Bus: Physical_Actuation
  Actuation Signals Out : PMIOPort  Port=6  Side=Right  ConnectionType=Bus: Physical_Actuation
  Multibody : PMIOPort  Port=7  Side=Right  ConnectionType=Bus: Physical_Multibody
  Bus Element Out1 : Outport  PortName=Measurements
  wires:
  Sensing/1 -> Impairments/1(Measurements In)
  Impairments/1(Measurements Out) -> Bus Element Out1/1
  connections:
  Sensing/RConn1 -- Motor Phases In/RConn1
  Sensing/RConn2 -- Motor Phases Out/RConn1
  Sensing/RConn3 -- Motors Signals In/RConn1
  Sensing/RConn4 -- Motors Signals Out/RConn1
  Sensing/RConn5 -- Actuation Signals In/RConn1
  Sensing/RConn6 -- Actuation Signals Out/RConn1
  Sensing/RConn7 -- Multibody/RConn1

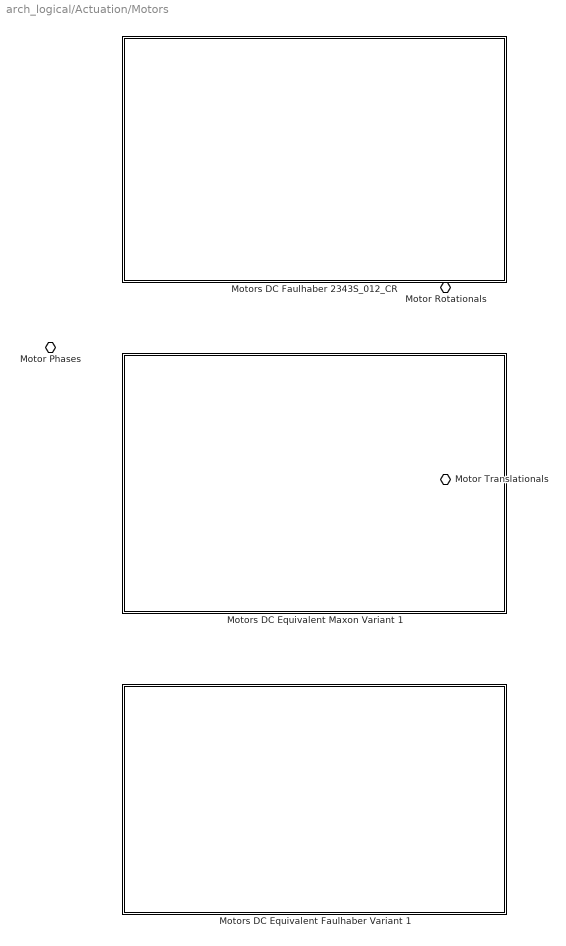
== system arch_logical/Actuation/Motors ==
  Motors DC Equivalent Faulhaber Variant 1 : Subsystem  VariantControl=Selector_Motor == Types_Motor.DCEquivalent_Faulhaber_Variant1  ReferencedSubsystem=MotorsDCEquivalentFaulhaber_Variant1
      settings: PermitHierarchicalResolution=None  PortSchema="{\"entries\":[{\"content\":{\"headerSize\":26,\"margin\":15,\"minimumSpacing\":25,\"sides\":[{\"content\":{\"connectorIds\":[\"LConn1\"]},\"type\":\"ConnectorPlacement.EquallySpacedRectSide\",\"uuid\":\"c73e21b5-dc95-496e-85f7-d918631fc64a\"},{\"content\":{\"connectorIds\":[\"RConn1\"],\"side\":\"RIGHT\"},\"type\":\"ConnectorPlacement.EquallySpacedRectSide\",\"uuid\":\"5236eb9f-21e4-4615-81a8-5c98c69e44ec\"},{\"content\":{\"side\":\"TOP\"},\"type\":\"ConnectorPlacement.EquallySpacedRectSide\",\"uuid\":\"362c231f-9a6d-4a83-afc1-2fbe43e23d2a\"}]},\"type\":\"ConnectorPlacement.EquallySpacedConnector\",\"uuid\":\"494d6a56-3818-488e-99cc-7df5051f7e30\"}],\"packageUris\":[\"http://schema.mathworks.com/mf0/Connector/R2020b\"],\"version\":\"1.0\"}"
  Motors DC Equivalent Maxon Variant 1 : Subsystem  VariantControl=Selector_Motor == Types_Motor.DCEquivalent_Maxon_Variant1  ReferencedSubsystem=MotorsDCEquivalentMaxon_Variant1
      settings: PermitHierarchicalResolution=None  PortSchema="{\"entries\":[{\"content\":{\"headerSize\":26,\"margin\":15,\"minimumSpacing\":25,\"sides\":[{\"content\":{\"connectorIds\":[\"LConn1\"]},\"type\":\"ConnectorPlacement.EquallySpacedRectSide\",\"uuid\":\"25b65f7d-f824-4ba3-b1ed-62665898e2af\"},{\"content\":{\"connectorIds\":[\"RConn1\"],\"side\":\"RIGHT\"},\"type\":\"ConnectorPlacement.EquallySpacedRectSide\",\"uuid\":\"9487a21d-3ba6-4fe2-bdba-f10d1b29e9d5\"},{\"content\":{\"side\":\"TOP\"},\"type\":\"ConnectorPlacement.EquallySpacedRectSide\",\"uuid\":\"4746a095-1b27-40e2-b199-adb40e90c46e\"}]},\"type\":\"ConnectorPlacement.EquallySpacedConnector\",\"uuid\":\"2d26b106-d6e1-4bff-b1c2-31dab5640331\"}],\"packageUris\":[\"http://schema.mathworks.com/mf0/Connector/R2020b\"],\"version\":\"1.0\"}"
  Motors DC Faulhaber 2343S_012_CR : Subsystem  VariantControl=Selector_Motor == Types_Motor.DC_Faulhaber_2342S_012_CR  ReferencedSubsystem=MotorsDCFaulhaber_2342S_012_CR
      settings: PermitHierarchicalResolution=None  PortSchema="{\"entries\":[{\"content\":{\"headerSize\":26,\"margin\":15,\"minimumSpacing\":25,\"sides\":[{\"content\":{\"connectorIds\":[\"LConn1\"]},\"type\":\"ConnectorPlacement.EquallySpacedRectSide\",\"uuid\":\"02771a66-d9bf-471a-9ef2-5f7974b9c9b2\"},{\"content\":{\"connectorIds\":[\"RConn1\"],\"side\":\"RIGHT\"},\"type\":\"ConnectorPlacement.EquallySpacedRectSide\",\"uuid\":\"3d8184d5-3986-4fbe-aa13-f688338869c5\"},{\"content\":{\"side\":\"TOP\"},\"type\":\"ConnectorPlacement.EquallySpacedRectSide\",\"uuid\":\"3757a264-4740-4c2c-912e-8b5e888f6b44\"}]},\"type\":\"ConnectorPlacement.EquallySpacedConnector\",\"uuid\":\"1270c383-6cbb-429f-84fb-1a50316b8aca\"}],\"packageUris\":[\"http://schema.mathworks.com/mf0/Connector/R2020b\"],\"version\":\"1.0\"}"
  Motor Phases : PMIOPort  Side=Left
  Motor Rotationals : PMIOPort  Port=2  Side=Right  ConnectionType=Bus: Physical_MotorRotationals
  Motor Translationals : PMIOPort  Port=3  Side=Right  ConnectionType=Bus: Physical_MotorTranslationals

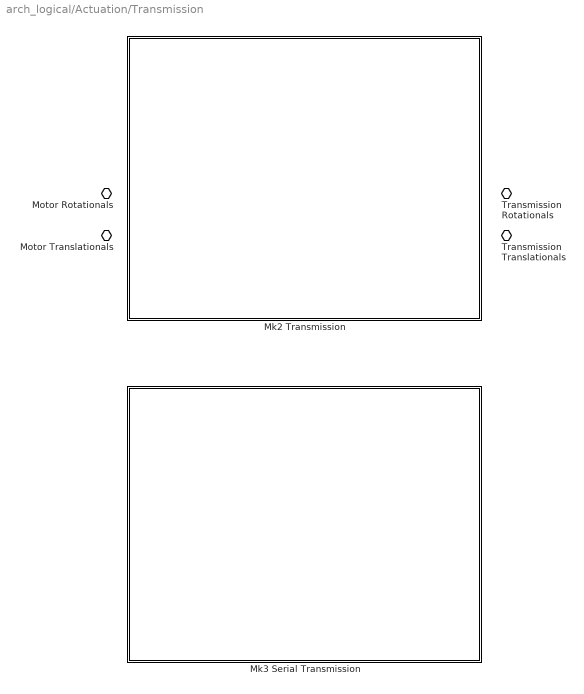
== system arch_logical/Actuation/Transmission ==
  Mk2 Transmission : Subsystem  VariantControl=Selector_Transmission == Types_Transmission.Mk2  ReferencedSubsystem=Mk2Transmission
      settings: PermitHierarchicalResolution=None  PortSchema="{\"entries\":[{\"content\":{\"headerSize\":26,\"margin\":15,\"minimumSpacing\":25,\"sides\":[{\"content\":{\"connectorIds\":[\"LConn1\"]},\"type\":\"ConnectorPlacement.EquallySpacedRectSide\",\"uuid\":\"eccd4d58-2367-4793-bf9f-2eede0847c93\"},{\"content\":{\"connectorIds\":[\"RConn1\"],\"side\":\"RIGHT\"},\"type\":\"ConnectorPlacement.EquallySpacedRectSide\",\"uuid\":\"32519a16-e586-4f6e-b8f0-36f1e508df36\"},{\"content\":{\"side\":\"TOP\"},\"type\":\"ConnectorPlacement.EquallySpacedRectSide\",\"uuid\":\"f22ee251-d4b1-48ea-b188-f62260b2e429\"}]},\"type\":\"ConnectorPlacement.EquallySpacedConnector\",\"uuid\":\"8d6616d9-e499-47c7-92ab-9373a8f1fb5b\"}],\"packageUris\":[\"http://schema.mathworks.com/mf0/Connector/R2020b\"],\"version\":\"1.0\"}"
  Mk3 Serial Transmission : Subsystem  VariantControl=Selector_Transmission == Types_Transmission.Mk3_Serial  ReferencedSubsystem=Mk3SerialTransmission
      settings: PermitHierarchicalResolution=None  PortSchema="{\"entries\":[{\"content\":{\"headerSize\":26,\"margin\":15,\"minimumSpacing\":25,\"sides\":[{\"content\":{\"connectorIds\":[\"LConn1\"]},\"type\":\"ConnectorPlacement.EquallySpacedRectSide\",\"uuid\":\"25b65f7d-f824-4ba3-b1ed-62665898e2af\"},{\"content\":{\"connectorIds\":[\"RConn1\"],\"side\":\"RIGHT\"},\"type\":\"ConnectorPlacement.EquallySpacedRectSide\",\"uuid\":\"9487a21d-3ba6-4fe2-bdba-f10d1b29e9d5\"},{\"content\":{\"side\":\"TOP\"},\"type\":\"ConnectorPlacement.EquallySpacedRectSide\",\"uuid\":\"4746a095-1b27-40e2-b199-adb40e90c46e\"}]},\"type\":\"ConnectorPlacement.EquallySpacedConnector\",\"uuid\":\"2d26b106-d6e1-4bff-b1c2-31dab5640331\"}],\"packageUris\":[\"http://schema.mathworks.com/mf0/Connector/R2020b\"],\"version\":\"1.0\"}"
  Transmission Rotationals : PMIOPort  Side=Right  ConnectionType=Bus: Physical_TransmissionRotationals
  Motor Rotationals : PMIOPort  Port=2  Side=Left  ConnectionType=Bus: Physical_MotorRotationals
  Motor Translationals : PMIOPort  Port=3  Side=Left  ConnectionType=Bus: Physical_MotorTranslationals
  Transmission Translationals : PMIOPort  Port=4  Side=Right  ConnectionType=Bus: Physical_TransmissionTranslationals

== system arch_logical/External Disturbances/None ==
  Bus Element In1 : Inport  PortName=Disturbances
  Terminator : Terminator
  Env1 : PMIOPort  Side=Left  ConnectionType=Bus: Physical_Environment
  Env2 : PMIOPort  Port=2  Side=Right  ConnectionType=Bus: Physical_Environment
  wires:
  Bus Element In1/1 -> Terminator/1
  connections:
  Env1/RConn1 -- Env2/RConn1

== system arch_logical/MCU/Controller ==
  Joint References : Inport  OutDataTypeStr=Bus: Data_JointReferences
  Control Feedback : Inport  Port=2  OutDataTypeStr=Bus: Data_ControlFeedback
  Mk2 Controller : Subsystem  VariantControl=Selector_Controller == Types_Controller.Mk2  ReferencedSubsystem=Mk2Controller
      settings: PermitHierarchicalResolution=None  PortSchema="{\"entries\":[{\"content\":{\"headerSize\":26,\"margin\":15,\"minimumSpacing\":25,\"sides\":[{\"content\":{\"connectorIds\":[\"In1\",\"In2\"]},\"type\":\"ConnectorPlacement.EquallySpacedRectSide\",\"uuid\":\"02771a66-d9bf-471a-9ef2-5f7974b9c9b2\"},{\"content\":{\"connectorIds\":[\"Out1\"],\"side\":\"RIGHT\"},\"type\":\"ConnectorPlacement.EquallySpacedRectSide\",\"uuid\":\"3d8184d5-3986-4fbe-aa13-f688338869c5\"},{\"content\":{\"side\":\"TOP\"},\"type\":\"ConnectorPlacement.EquallySpacedRectSide\",\"uuid\":\"3757a264-4740-4c2c-912e-8b5e888f6b44\"}]},\"type\":\"ConnectorPlacement.EquallySpacedConnector\",\"uuid\":\"1270c383-6cbb-429f-84fb-1a50316b8aca\"}],\"packageUris\":[\"http://schema.mathworks.com/mf0/Connector/R2020b\"],\"version\":\"1.0\"}"
  Mk3 Serial Controller : Subsystem  VariantControl=Selector_Controller == Types_Controller.Mk3_Serial  ReferencedSubsystem=Mk3SerialController
      settings: PermitHierarchicalResolution=None  PortSchema="{\"entries\":[{\"content\":{\"headerSize\":26,\"margin\":15,\"minimumSpacing\":25,\"sides\":[{\"content\":{\"connectorIds\":[\"In1\",\"In2\"]},\"type\":\"ConnectorPlacement.EquallySpacedRectSide\",\"uuid\":\"25b65f7d-f824-4ba3-b1ed-62665898e2af\"},{\"content\":{\"connectorIds\":[\"Out1\"],\"side\":\"RIGHT\"},\"type\":\"ConnectorPlacement.EquallySpacedRectSide\",\"uuid\":\"9487a21d-3ba6-4fe2-bdba-f10d1b29e9d5\"},{\"content\":{\"side\":\"TOP\"},\"type\":\"ConnectorPlacement.EquallySpacedRectSide\",\"uuid\":\"4746a095-1b27-40e2-b199-adb40e90c46e\"}]},\"type\":\"ConnectorPlacement.EquallySpacedConnector\",\"uuid\":\"2d26b106-d6e1-4bff-b1c2-31dab5640331\"}],\"packageUris\":[\"http://schema.mathworks.com/mf0/Connector/R2020b\"],\"version\":\"1.0\"}"
  Commands : Outport  OutDataTypeStr=Bus: Data_ControlCommands

== system arch_logical/MCU/Planner ==
  Joint References In : Inport
  Planner MinJerk : Subsystem  VariantControl=Selector_Planner == Types_Planner.MinJerk  ReferencedSubsystem=PlannerMinJerk
      settings: PermitHierarchicalResolution=None  PortSchema="{\"entries\":[{\"content\":{\"headerSize\":26,\"margin\":15,\"minimumSpacing\":25,\"sides\":[{\"content\":{\"connectorIds\":[\"In1\"]},\"type\":\"ConnectorPlacement.EquallySpacedRectSide\",\"uuid\":\"4bb9fa66-7008-4226-909e-fef797898c3d\"},{\"content\":{\"connectorIds\":[\"Out1\"],\"side\":\"RIGHT\"},\"type\":\"ConnectorPlacement.EquallySpacedRectSide\",\"uuid\":\"9a6ed126-9c10-4aa4-84eb-0818ed759a08\"},{\"content\":{\"side\":\"TOP\"},\"type\":\"ConnectorPlacement.EquallySpacedRectSide\",\"uuid\":\"bb6df1d3-ee30-41ba-9c4f-73e73f4c287f\"}]},\"type\":\"ConnectorPlacement.EquallySpacedConnector\",\"uuid\":\"87603bc8-7dd7-4df2-b4ba-c705ac93164f\"}],\"packageUris\":[\"http://schema.mathworks.com/mf0/Connector/R2020b\"],\"version\":\"1.0\"}"
  Planner None : Subsystem  VariantControl=Selector_Planner == Types_Planner.None
      settings: PortSchema="{\"entries\":[{\"content\":{\"headerSize\":26,\"margin\":15,\"minimumSpacing\":25,\"sides\":[{\"content\":{\"connectorIds\":[\"In1\"]},\"type\":\"ConnectorPlacement.EquallySpacedRectSide\",\"uuid\":\"4dcdf3d9-66d1-4b2d-9c68-f21e4e282afd\"},{\"content\":{\"connectorIds\":[\"Out1\"],\"side\":\"RIGHT\"},\"type\":\"ConnectorPlacement.EquallySpacedRectSide\",\"uuid\":\"3179edab-f19d-4e86-a6d0-5fab8993b041\"},{\"content\":{\"side\":\"TOP\"},\"type\":\"ConnectorPlacement.EquallySpacedRectSide\",\"uuid\":\"71bb34ca-738a-4841-9245-23739004f511\"}]},\"type\":\"ConnectorPlacement.EquallySpacedConnector\",\"uuid\":\"4120f61b-053a-45ce-ab11-ff3b69017e22\"}],\"packageUris\":[\"http://schema.mathworks.com/mf0/Connector/R2020b\"],\"version\":\"1.0\"}"
  Joint References Out : Outport

== system arch_logical/MCU/Signal Processing ==
  Measurements : Inport
  Signal Processing None : Subsystem  VariantControl=Selector_SignalProcessing == Types_SignalProcessing.None
      settings: PortSchema="{\"entries\":[{\"content\":{\"headerSize\":26,\"margin\":15,\"minimumSpacing\":25,\"sides\":[{\"content\":{\"connectorIds\":[\"In1\"]},\"type\":\"ConnectorPlacement.EquallySpacedRectSide\",\"uuid\":\"eccd4d58-2367-4793-bf9f-2eede0847c93\"},{\"content\":{\"connectorIds\":[\"Out1\"],\"side\":\"RIGHT\"},\"type\":\"ConnectorPlacement.EquallySpacedRectSide\",\"uuid\":\"32519a16-e586-4f6e-b8f0-36f1e508df36\"},{\"content\":{\"side\":\"TOP\"},\"type\":\"ConnectorPlacement.EquallySpacedRectSide\",\"uuid\":\"f22ee251-d4b1-48ea-b188-f62260b2e429\"},{\"content\":{\"side\":\"BOTTOM\"},\"type\":\"ConnectorPlacement.EquallySpacedRectSide\",\"uuid\":\"044c0013-73b4-4eb7-b0dc-011a4b3384d3\"}]},\"type\":\"ConnectorPlacement.EquallySpacedConnector\",\"uuid\":\"8d6616d9-e499-47c7-92ab-9373a8f1fb5b\"}],\"packageUris\":[\"http://schema.mathworks.com/mf0/Connector/R2020b\"],\"version\":\"1.0\"}"
  Control Feedback : Outport
